simulink model "old_prova_ottimale"  (R2024a)
settings: Solver=VariableStepAuto  StartTime=0.0  StopTime=3000  RelTol=1e-3
undefined symbols (not defined in the file): cp, pitch, TSR
libraries: simulink x4, spsDCMachineLib x1, spsVoltageMeasurementLib x1, sps_lib x1
settings Model: Creator=emanuele  LastModifiedBy=emanuele

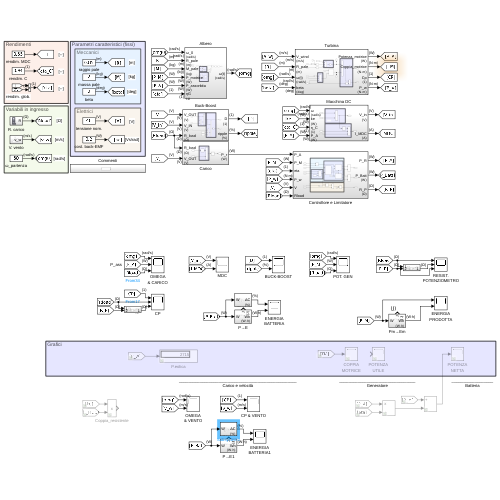
[thumbnail: Simulink's stored preview of the top-level diagram]
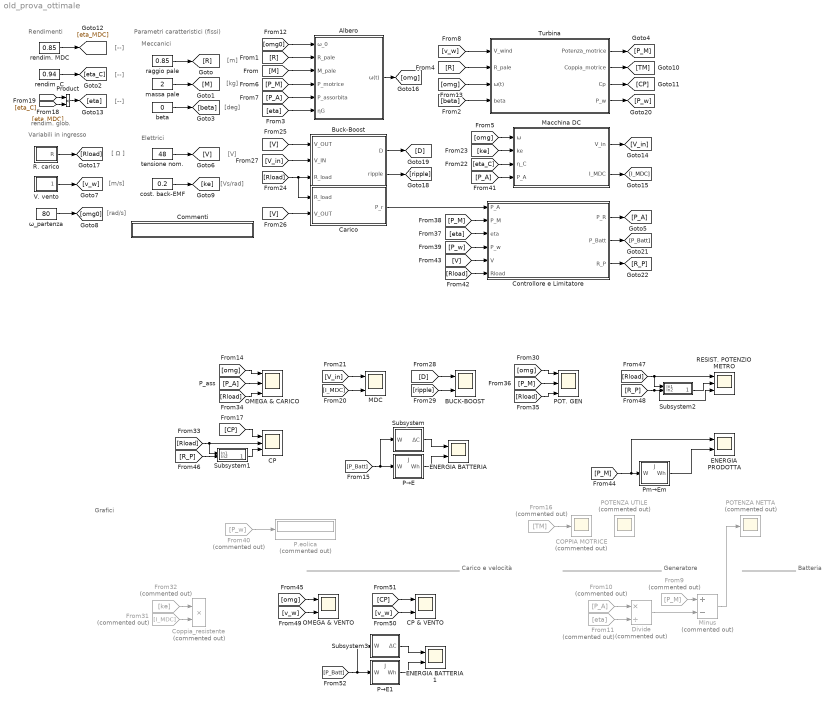
== system old_prova_ottimale ==
  note: rendim. glob.
  note: ___________________________________________________
      | Carico e velocità
  note: Elettrici
  note: Meccanici
  note: Grafici
  note: Variabili in ingresso
  note: [m]
  note: Parametri caratteristici (fissi)
  note: [kg]
  note: [deg]
  note: [ Ω ]
  note: [V]
  note: [m/s]
  note: _________________________________
      | Generatore
  note: __________________
      | Batteria
  note: [rad/s]
  note: Rendimenti
  note: [--]
  note: [--]
  note: [--]
  note: [Vs/rad]
  Albero : Subsystem
  BUCK-BOOST : Scope  NumInputPorts=2
  Buck-Boost : Subsystem
  COPPIA MOTRICE : Scope  Commented=on
  CP : Scope  NumInputPorts=3
  CP & VENTO : Scope  NumInputPorts=2
  Carico : Subsystem
  Commenti : Subsystem
  Controllore e Limitatore : Subsystem
  Coppia_resistente : Product  Commented=on
  Divide : Product  Commented=on  Inputs=*/
  ENERGIA BATTERIA : Scope  NumInputPorts=2
  ENERGIA BATTERIA1 : Scope  NumInputPorts=2
  ENERGIA PRODOTTA : Scope  NumInputPorts=2
  From10 : From  Commented=on  GotoTag=P_A
  From11 : From  Commented=on  GotoTag=eta
  From16 : From  Commented=on  GotoTag=TM
  From31 : From  Commented=on  GotoTag=I_MDC
  From32 : From  Commented=on  GotoTag=ke
  From40 : From  Commented=on  GotoTag=P_w
  From9 : From  Commented=on  GotoTag=P_M
  MDC : Scope  NumInputPorts=2
  Macchina DC : Subsystem
  Minus : Sum  Commented=on  Inputs=+-
  OMEGA & CARICO : Scope  NumInputPorts=3
  OMEGA & VENTO : Scope  NumInputPorts=2
  P.eolica : Display  Commented=on
  POT. GEN : Scope  NumInputPorts=3
  POTENZA NETTA : Scope  Commented=on
  POTENZA UTILE : Scope  Commented=on
  Pm→Em : Subsystem
      settings: PortSchema="{\"entries\":[{\"content\":{\"sides\":[{\"content\":{\"connectorIds\":[\"In1\"]},\"type\":\"ConnectorPlacement.EquallySpacedRectSide\",\"uuid\":\"bcdc19f3-31c9-4960-9b75-9687f3be57dc\"},{\"content\":{\"connectorIds\":[\"Out1\"],\"side\":\"RIGHT\"},\"type\":\"ConnectorPlacement.EquallySpacedRectSide\",\"uuid\":\"6f4d4c58-42a6-48b0-9f12-2aa1dcddf363\"},{\"content\":{\"connectorIds\":[\"Out2\"],\"side\":\"TOP\"},\"type\":\"ConnectorPlacement.EquallySpacedRectSide\",\"uuid\":\"abeed6e6-3a12-4b7a-a1c3-2526a61f695c\"},{\"content\":{\"side\":\"BOTTOM\"},\"type\":\"ConnectorPlacement.EquallySpacedRectSide\",\"uuid\":\"4f3a7421-d380-4df7-a1ed-c17c06ed2066\"}]},\"type\":\"ConnectorPlacement.EquallySpacedConnector\",\"uuid\":\"402fec35-a9bf-47fd-aac8-c2826b6cf801\"}],\"packageUris\":[\"http://schema.mathworks.com/mf0/Connector/R2020b\"],\"version\":\"1.0\"}"
  Product : Product
  P→E : Subsystem
      settings: PortSchema="{\"entries\":[{\"content\":{\"sides\":[{\"content\":{\"connectorIds\":[\"In1\"]},\"type\":\"ConnectorPlacement.EquallySpacedRectSide\",\"uuid\":\"bcdc19f3-31c9-4960-9b75-9687f3be57dc\"},{\"content\":{\"connectorIds\":[\"Out1\"],\"side\":\"RIGHT\"},\"type\":\"ConnectorPlacement.EquallySpacedRectSide\",\"uuid\":\"6f4d4c58-42a6-48b0-9f12-2aa1dcddf363\"},{\"content\":{\"connectorIds\":[\"Out2\"],\"side\":\"TOP\"},\"type\":\"ConnectorPlacement.EquallySpacedRectSide\",\"uuid\":\"abeed6e6-3a12-4b7a-a1c3-2526a61f695c\"},{\"content\":{\"side\":\"BOTTOM\"},\"type\":\"ConnectorPlacement.EquallySpacedRectSide\",\"uuid\":\"4f3a7421-d380-4df7-a1ed-c17c06ed2066\"}]},\"type\":\"ConnectorPlacement.EquallySpacedConnector\",\"uuid\":\"402fec35-a9bf-47fd-aac8-c2826b6cf801\"}],\"packageUris\":[\"http://schema.mathworks.com/mf0/Connector/R2020b\"],\"version\":\"1.0\"}"
  P→E1 : Subsystem
      settings: PortSchema="{\"entries\":[{\"content\":{\"sides\":[{\"content\":{\"connectorIds\":[\"In1\"]},\"type\":\"ConnectorPlacement.EquallySpacedRectSide\",\"uuid\":\"bcdc19f3-31c9-4960-9b75-9687f3be57dc\"},{\"content\":{\"connectorIds\":[\"Out1\"],\"side\":\"RIGHT\"},\"type\":\"ConnectorPlacement.EquallySpacedRectSide\",\"uuid\":\"6f4d4c58-42a6-48b0-9f12-2aa1dcddf363\"},{\"content\":{\"connectorIds\":[\"Out2\"],\"side\":\"TOP\"},\"type\":\"ConnectorPlacement.EquallySpacedRectSide\",\"uuid\":\"abeed6e6-3a12-4b7a-a1c3-2526a61f695c\"},{\"content\":{\"side\":\"BOTTOM\"},\"type\":\"ConnectorPlacement.EquallySpacedRectSide\",\"uuid\":\"4f3a7421-d380-4df7-a1ed-c17c06ed2066\"}]},\"type\":\"ConnectorPlacement.EquallySpacedConnector\",\"uuid\":\"402fec35-a9bf-47fd-aac8-c2826b6cf801\"}],\"packageUris\":[\"http://schema.mathworks.com/mf0/Connector/R2020b\"],\"version\":\"1.0\"}"
  R. carico : Subsystem
  RESIST. POTENZIOMETRO : Scope  NumInputPorts=3
  Subsystem : Subsystem
  Subsystem1 : Subsystem
  Subsystem2 : Subsystem
  Subsystem3 : Subsystem
  Turbina : Subsystem
  V. vento : Subsystem
  beta : Constant  Value=0
  cost. back-EMF : Constant  Value=0.2
  massa pale : Constant  Value=2
  raggio pale : Constant  Value=0.85
  rendim. C : Constant  Value=0.94
  rendim. MDC : Constant  Value=0.85
  tensione nom. : Constant  Value=48
  ω_partenza : Constant  Value=80
  wires:
  raggio pale/1 -> [R]
  massa pale/1 -> [M]
  beta/1 -> [beta]
  [R] -> Albero/2(R_pale)
  [M] -> Albero/3(M_pale)
  [beta] -> Turbina/4(beta)
  [eta] -> Albero/6(ηG)
  [R] -> Turbina/2(R_pale)
  [P_M] -> Albero/4(P_motrice)
  [P_A] -> Albero/5(P_assorbita)
  tensione nom./1 -> [V]
  [P_A] -> OMEGA & CARICO/2
  [v_w] -> Turbina/1(V_wind)
  From9/1 -> Minus/1
  Minus/1 -> POTENZA NETTA/1
  From11/1 -> Divide/2
  From10/1 -> Divide/1
  Divide/1 -> Minus/2
  V. vento/1(v_w) -> [v_w]
  ω_partenza/1 -> [omg0]
  [omg0] -> Albero/1(ω_0)
  Albero/1(ω(t)) -> [omg]
  [omg] -> Macchina DC/1(ω)
  [omg] -> Turbina/3(ω(t))
  [omg] -> OMEGA & CARICO/1
  Turbina/1(Potenza_motrice) -> [P_M]
  [P_Batt] -> Subsystem/1(W), P→E/1(W)
  Turbina/2(Coppia_motrice) -> [TM]
  From16/1 -> COPPIA MOTRICE/1
  Turbina/3(Cp) -> [CP]
  rendim. MDC/1 -> [eta_MDC]
  rendim. C/1 -> [eta_C]
  Product/1 -> [eta]
  [eta_MDC] -> Product/1
  [eta_C] -> Product/2
  [eta_C] -> Macchina DC/3(η_C)
  Macchina DC/1(V_in) -> [V_in]
  Macchina DC/2(I_MDC) -> [I_MDC]
  [V_in] -> MDC/1
  [I_MDC] -> MDC/2
  cost. back-EMF/1 -> [ke]
  [ke] -> Macchina DC/2(ke)
  R. carico/1(R) -> [Rload]
  [Rload] -> Carico/1(R_load), Buck-Boost/3(R_load)
  [V] -> Buck-Boost/1(V_OUT)
  [V] -> Carico/2(V_OUT)
  [V_in] -> Buck-Boost/2(V_IN)
  Buck-Boost/2(ripple) -> [ripple]
  Buck-Boost/1(D) -> [D]
  [D] -> BUCK-BOOST/1
  [ripple] -> BUCK-BOOST/2
  From31/1 -> Coppia_resistente/2
  From32/1 -> Coppia_resistente/1
  [Rload] -> OMEGA & CARICO/3
  [omg] -> POT. GEN/1
  [Rload] -> POT. GEN/3
  [P_M] -> POT. GEN/2
  Carico/1(P_r) -> Controllore e Limitatore/1(P_A)
  Controllore e Limitatore/1(P_R) -> [P_A]
  [P_M] -> Controllore e Limitatore/2(P_M)
  [eta] -> Controllore e Limitatore/3(eta)
  Turbina/4(P_w) -> [P_w]
  [P_w] -> Controllore e Limitatore/4(P_w)
  From40/1 -> P.eolica/1
  Controllore e Limitatore/2(P_Batt) -> [P_Batt]
  [P_A] -> Macchina DC/4(P_A)
  [V] -> Controllore e Limitatore/5(V)
  [Rload] -> Controllore e Limitatore/6(Rload)
  Controllore e Limitatore/3(R_P) -> [R_P]
  [CP] -> CP/1
  [Rload] -> CP/2, Subsystem1/1(In1)
  [R_P] -> Subsystem1/2(In2)
  Subsystem1/1(Out1) -> CP/3
  Subsystem2/1(Out1) -> RESIST. POTENZIOMETRO/2
  [R_P] -> RESIST. POTENZIOMETRO/3, Subsystem2/2(In2)
  [Rload] -> RESIST. POTENZIOMETRO/1, Subsystem2/1(In1)
  [P_M] -> ENERGIA PRODOTTA/1, Pm→Em/1(W)
  Pm→Em/1(Wh) -> ENERGIA PRODOTTA/2
  Subsystem/1(ΔC) -> ENERGIA BATTERIA/1
  P→E/1(Wh) -> ENERGIA BATTERIA/2
  [omg] -> OMEGA & VENTO/1
  [v_w] -> OMEGA & VENTO/2
  [v_w] -> CP & VENTO/2
  [CP] -> CP & VENTO/1
  P→E1/1(Wh) -> ENERGIA BATTERIA1/2
  Subsystem3/1(ΔC) -> ENERGIA BATTERIA1/1
  [P_Batt] -> P→E1/1(W), Subsystem3/1(W)

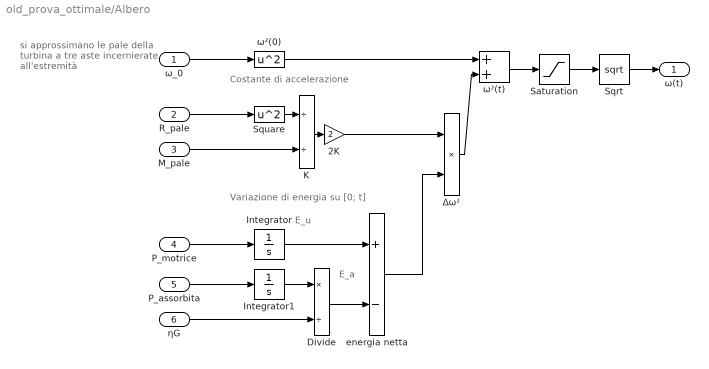
== system old_prova_ottimale/Albero ==
  note: Costante di accelerazione
  note: Variazione di energia su [0; t]
  note: si approssimano le pale
      | della turbina a tre aste
      | incernierate all'estremità
  note: E_a
  note: E_u
  ω_0 : Inport  Unit=rad/s
  R_pale : Inport  Port=2  Unit=m
  M_pale : Inport  Port=3  Unit=kg
  P_motrice : Inport  Port=4  Unit=W
  P_assorbita : Inport  Port=5  Unit=W
  ηG : Inport  Port=6  Unit=1
  2K : Gain  Gain=2
  Divide : Product  Inputs=*/
  Integrator : Integrator
  Integrator1 : Integrator
  K : Product  Inputs=//
  Saturation : Saturate  UpperLimit=10e6  LowerLimit=0
  Sqrt : Sqrt
  Square : Math  Operator=square
  energia netta : Sum  Inputs=+-
  Δω² : Product
  ω²(0) : Math  Operator=square
  ω²(t) : Sum
  ω(t) : Outport  Unit=rad/s
  wires:
  M_pale/1 -> K/2
  K/1 -> 2K/1
  Sqrt/1 -> ω(t)/1
  energia netta/1 -> Δω²/2
  Integrator/1 -> energia netta/1
  R_pale/1 -> Square/1
  P_assorbita/1 -> Integrator1/1
  Integrator1/1 -> Divide/1
  Δω²/1 -> ω²(t)/2
  Square/1 -> K/1
  P_motrice/1 -> Integrator/1
  ω²(0)/1 -> ω²(t)/1
  ω_0/1 -> ω²(0)/1
  ω²(t)/1 -> Saturation/1
  2K/1 -> Δω²/1
  Divide/1 -> energia netta/2
  ηG/1 -> Divide/2
  Saturation/1 -> Sqrt/1

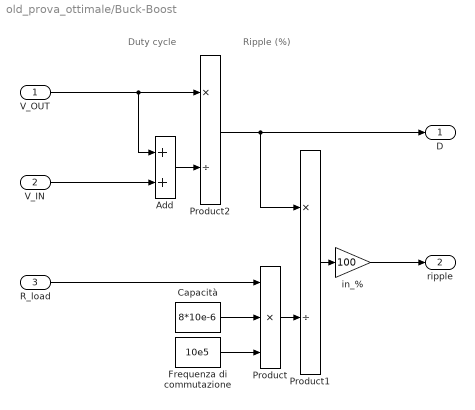
== system old_prova_ottimale/Buck-Boost ==
  note: Duty cycle
  note: Ripple (%)
  V_OUT : Inport  Unit=V
  V_IN : Inport  Port=2  Unit=V
  R_load : Inport  Port=3  Unit=Ω
  Add : Sum
  Capacità : Constant  Value=8*10e-6
  Frequenza di commutazione : Constant  Value=10e5
  Product : Product  Inputs=3
  Product1 : Product  Inputs=*/
  Product2 : Product  Inputs=*/
  in_% : Gain  Gain=100
  D : Outport  Unit=1
  ripple : Outport  Port=2  Unit=%
  wires:
  R_load/1 -> Product/1
  Capacità/1 -> Product/2
  V_IN/1 -> Add/2
  Frequenza di commutazione/1 -> Product/3
  Product/1 -> Product1/2
  V_OUT/1 -> Product2/1, Add/1
  Add/1 -> Product2/2
  Product1/1 -> in_%/1
  in_%/1 -> ripple/1
  Product2/1 -> D/1, Product1/1

== system old_prova_ottimale/Carico ==
  note: Carico
  R_load : Inport  Unit=Ω
  V_OUT : Inport  Port=2  Unit=V
  Product : Product  Inputs=*/
  Saturation : Saturate  UpperLimit=10e6  LowerLimit=0.1
  Square : Math  Operator=square
  P_r : Outport  Unit=W
  wires:
  Square/1 -> Product/1
  R_load/1 -> Product/2
  Product/1 -> Saturation/1
  V_OUT/1 -> Square/1
  Saturation/1 -> P_r/1

== system old_prova_ottimale/Commenti ==
  note: % se omega = 0 → solo P_A
      | % come calcolo il deficit di energia?
  vecchia MDC : Subsystem  Commented=on

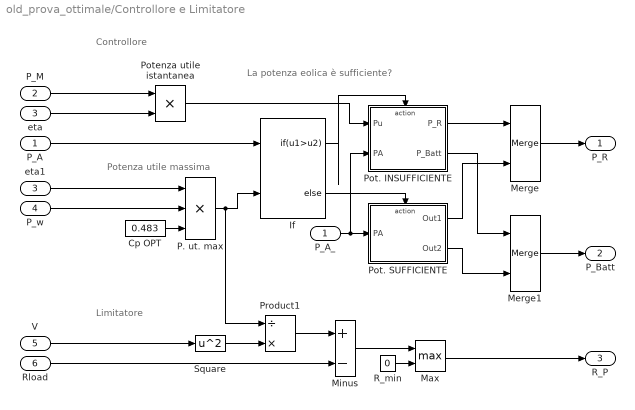
== system old_prova_ottimale/Controllore e Limitatore ==
  note: Limitatore
  note: Controllore
  note: Potenza utile massima
  note: La potenza eolica è sufficiente?
  P_A : Inport
  P_M : Inport  Port=2
  eta : Inport  Port=3
  P_w : Inport  Port=4
  V : Inport  Port=5
  Rload : Inport  Port=6
  Cp OPT : Constant  Value=0.483
  If : If  NumInputs=2  IfExpression=u1>u2
  Max : MinMax  Function=max  Inputs=2
  Merge : Merge
  Merge1 : Merge
  Minus : Sum  Inputs=+-
  P. ut. max : Product  Inputs=3
  P_A_ : InportShadow
  Pot. INSUFFICIENTE : Subsystem  TreatAsAtomicUnit=on
  Pot. SUFFICIENTE : Subsystem  TreatAsAtomicUnit=on
  Potenza utile istantanea : Product
  Product1 : Product  Inputs=/*
  R_min : Constant  Value=0
  Square : Math  Operator=square
  eta1 : InportShadow  Port=3
  P_R : Outport
  P_Batt : Outport  Port=2  Unit=W
  R_P : Outport  Port=3  Unit=Ω
  wires:
  P_M/1 -> Potenza utile istantanea/1
  eta/1 -> Potenza utile istantanea/2
  Pot. SUFFICIENTE/1(Out1) -> Merge/2
  Merge/1 -> P_R/1
  Pot. INSUFFICIENTE/1(P_R) -> Merge/1
  If/2 -> Pot. SUFFICIENTE/Action
  P_A/1 -> If/1
  Potenza utile istantanea/1 -> Pot. INSUFFICIENTE/1(Pu)
  P_A_/1 -> Pot. INSUFFICIENTE/2(PA), Pot. SUFFICIENTE/1(PA)
  If/1 -> Pot. INSUFFICIENTE/Action
  eta1/1 -> P. ut. max/1
  P_w/1 -> P. ut. max/2
  Cp OPT/1 -> P. ut. max/3
  Merge1/1 -> P_Batt/1
  Pot. SUFFICIENTE/2(Out2) -> Merge1/2
  Pot. INSUFFICIENTE/2(P_Batt) -> Merge1/1
  V/1 -> Square/1
  Square/1 -> Product1/2
  Product1/1 -> Minus/1
  Rload/1 -> Minus/2
  Max/1 -> R_P/1
  Minus/1 -> Max/1
  R_min/1 -> Max/2
  P. ut. max/1 -> Product1/1, If/2

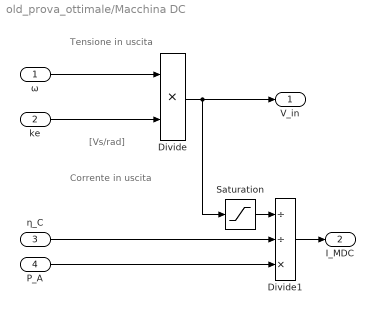
== system old_prova_ottimale/Macchina DC ==
  note: Corrente in uscita
  note: [Vs/rad]
  note: Tensione in uscita
  ω : Inport  Unit=rad/s
  ke : Inport  Port=2  Unit=W
  η_C : Inport  Port=3  Unit=1
  P_A : Inport  Port=4  Unit=W
  Divide : Product
  Divide1 : Product  Inputs=//*
  Saturation : Saturate  UpperLimit=1000  LowerLimit=1
  V_in : Outport  Unit=V
  I_MDC : Outport  Port=2  Unit=A
  wires:
  ke/1 -> Divide/2
  η_C/1 -> Divide1/2
  Saturation/1 -> Divide1/1
  Divide1/1 -> I_MDC/1
  ω/1 -> Divide/1
  Divide/1 -> V_in/1, Saturation/1
  P_A/1 -> Divide1/3

== system old_prova_ottimale/Pm→Em ==
  W : Inport
  J→Wh : Gain  Gain=1/3600
  integrale in dt : Integrator
  Wh : Outport  Unit=W*h
  J : Outport  Port=2  Unit=J
  wires:
  integrale in dt/1 -> J/1, J→Wh/1
  J→Wh/1 -> Wh/1
  W/1 -> integrale in dt/1

== system old_prova_ottimale/P→E ==
  W : Inport
  Gain : Gain  Gain=-1
  J→Wh : Gain  Gain=1/3600
  integrale in dt : Integrator
  Wh : Outport  Unit=W*h
  J : Outport  Port=2  Unit=J
  wires:
  integrale in dt/1 -> Gain/1
  J→Wh/1 -> Wh/1
  W/1 -> integrale in dt/1
  Gain/1 -> J/1, J→Wh/1

== system old_prova_ottimale/P→E1 ==
  W : Inport
  Gain : Gain
  J→Wh : Gain  Gain=1/3600
  integrale in dt : Integrator
  Wh : Outport  Unit=W*h
  J : Outport  Port=2  Unit=J
  wires:
  Gain/1 -> J→Wh/1, J/1
  W/1 -> integrale in dt/1
  J→Wh/1 -> Wh/1
  integrale in dt/1 -> Gain/1

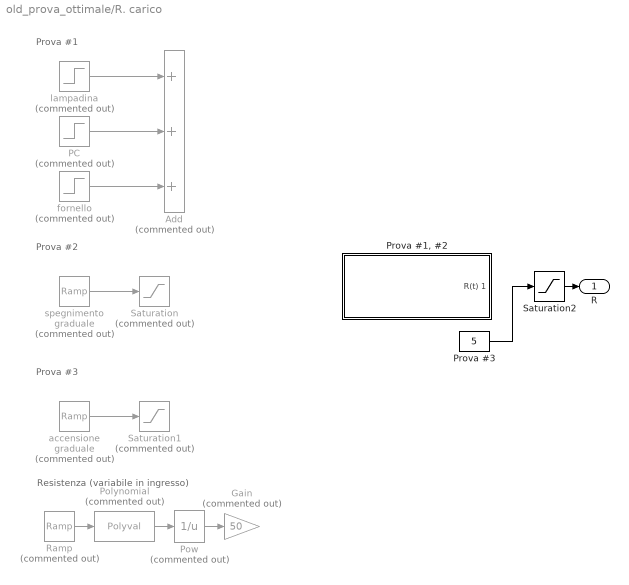
== system old_prova_ottimale/R. carico ==
  note: Prova #1
  note: Prova #2
  note: Prova #3
  note: Resistenza (variabile in ingresso)
  Add : Sum  Commented=on  Inputs=+++
  Gain : Gain  Commented=on  Gain=50
  PC : Step  Commented=on  Time=1200  After=90  SampleTime=0
  Polynomial : Polyval  Commented=on  Coefs=[10e-4 0 0]
  Pow : Math  Commented=on  Operator=reciprocal  SignedPower=on  RndMeth=Zero
  "Prova #1, #2" : Subsystem
  Prova #3 : Constant  Value=5
  Ramp : simulink/Sources/Ramp  Commented=on  slope=0.12  start=100  InitialOutput=0.1
  Saturation : Saturate  Commented=on  UpperLimit=1000  LowerLimit=0
  Saturation1 : Saturate  Commented=on  UpperLimit=200  LowerLimit=0
  Saturation2 : Saturate  UpperLimit=10e6  LowerLimit=0.15
  accensione graduale : simulink/Sources/Ramp  Commented=on  slope=2  start=900  InitialOutput=0
  fornello : Step  Commented=on  Time=1500  After=900  SampleTime=0
  lampadina : Step  Commented=on  Time=900  After=10  SampleTime=0
  spegnimento graduale : simulink/Sources/Ramp  Commented=on  slope=-10  start=900  InitialOutput=1000
  R : Outport
  wires:
  lampadina/1 -> Add/1
  PC/1 -> Add/2
  fornello/1 -> Add/3
  spegnimento graduale/1 -> Saturation/1
  accensione graduale/1 -> Saturation1/1
  Pow/1 -> Gain/1
  Ramp/1 -> Polynomial/1
  Polynomial/1 -> Pow/1
  Saturation2/1 -> R/1
  Prova #3/1 -> Saturation2/1

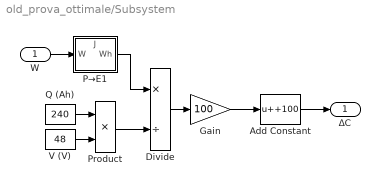
== system old_prova_ottimale/Subsystem ==
  W : Inport
  Add Constant : Bias  Bias=+100  SaturateOnIntegerOverflow=off
  Divide : Product  Inputs=*/
  Gain : Gain  Gain=100
  Product : Product
  P→E1 : Subsystem
      settings: PortSchema="{\"entries\":[{\"content\":{\"sides\":[{\"content\":{\"connectorIds\":[\"In1\"]},\"type\":\"ConnectorPlacement.EquallySpacedRectSide\",\"uuid\":\"bcdc19f3-31c9-4960-9b75-9687f3be57dc\"},{\"content\":{\"connectorIds\":[\"Out1\"],\"side\":\"RIGHT\"},\"type\":\"ConnectorPlacement.EquallySpacedRectSide\",\"uuid\":\"6f4d4c58-42a6-48b0-9f12-2aa1dcddf363\"},{\"content\":{\"connectorIds\":[\"Out2\"],\"side\":\"TOP\"},\"type\":\"ConnectorPlacement.EquallySpacedRectSide\",\"uuid\":\"abeed6e6-3a12-4b7a-a1c3-2526a61f695c\"},{\"content\":{\"side\":\"BOTTOM\"},\"type\":\"ConnectorPlacement.EquallySpacedRectSide\",\"uuid\":\"4f3a7421-d380-4df7-a1ed-c17c06ed2066\"}]},\"type\":\"ConnectorPlacement.EquallySpacedConnector\",\"uuid\":\"402fec35-a9bf-47fd-aac8-c2826b6cf801\"}],\"packageUris\":[\"http://schema.mathworks.com/mf0/Connector/R2020b\"],\"version\":\"1.0\"}"
  Q (Ah) : Constant  Value=240
  V (V) : Constant  Value=48
  ΔC : Outport  Unit=%
  wires:
  W/1 -> P→E1/1(W)
  V (V)/1 -> Product/2
  Q (Ah)/1 -> Product/1
  Product/1 -> Divide/2
  Divide/1 -> Gain/1
  P→E1/1(Wh) -> Divide/1
  Gain/1 -> Add Constant/1
  Add Constant/1 -> ΔC/1

== system old_prova_ottimale/Subsystem1 ==
  In1 : Inport
  In2 : Inport  Port=2
  Add : Sum
  Out1 : Outport  Unit=Ω
  wires:
  Add/1 -> Out1/1
  In2/1 -> Add/2
  In1/1 -> Add/1

== system old_prova_ottimale/Subsystem2 ==
  In1 : Inport
  In2 : Inport  Port=2
  Add : Sum
  Out1 : Outport  Unit=Ω
  wires:
  In1/1 -> Add/1
  In2/1 -> Add/2
  Add/1 -> Out1/1

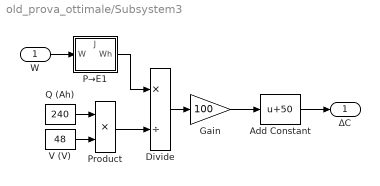
== system old_prova_ottimale/Subsystem3 ==
  W : Inport
  Add Constant : Bias  Bias=50  SaturateOnIntegerOverflow=off
  Divide : Product  Inputs=*/
  Gain : Gain  Gain=100
  Product : Product
  P→E1 : Subsystem
      settings: PortSchema="{\"entries\":[{\"content\":{\"sides\":[{\"content\":{\"connectorIds\":[\"In1\"]},\"type\":\"ConnectorPlacement.EquallySpacedRectSide\",\"uuid\":\"bcdc19f3-31c9-4960-9b75-9687f3be57dc\"},{\"content\":{\"connectorIds\":[\"Out1\"],\"side\":\"RIGHT\"},\"type\":\"ConnectorPlacement.EquallySpacedRectSide\",\"uuid\":\"6f4d4c58-42a6-48b0-9f12-2aa1dcddf363\"},{\"content\":{\"connectorIds\":[\"Out2\"],\"side\":\"TOP\"},\"type\":\"ConnectorPlacement.EquallySpacedRectSide\",\"uuid\":\"abeed6e6-3a12-4b7a-a1c3-2526a61f695c\"},{\"content\":{\"side\":\"BOTTOM\"},\"type\":\"ConnectorPlacement.EquallySpacedRectSide\",\"uuid\":\"4f3a7421-d380-4df7-a1ed-c17c06ed2066\"}]},\"type\":\"ConnectorPlacement.EquallySpacedConnector\",\"uuid\":\"402fec35-a9bf-47fd-aac8-c2826b6cf801\"}],\"packageUris\":[\"http://schema.mathworks.com/mf0/Connector/R2020b\"],\"version\":\"1.0\"}"
  Q (Ah) : Constant  Value=240
  V (V) : Constant  Value=48
  ΔC : Outport  Unit=%
  wires:
  Add Constant/1 -> ΔC/1
  Gain/1 -> Add Constant/1
  P→E1/1(Wh) -> Divide/1
  Divide/1 -> Gain/1
  Product/1 -> Divide/2
  Q (Ah)/1 -> Product/1
  V (V)/1 -> Product/2
  W/1 -> P→E1/1(W)

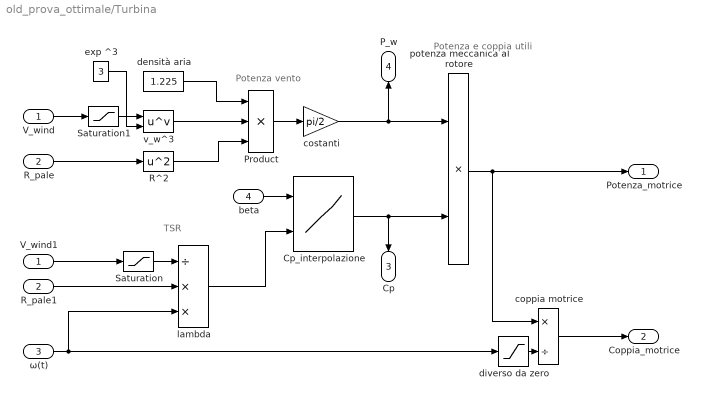
== system old_prova_ottimale/Turbina ==
  note: Potenza e coppia utili
  note: TSR
  note: Potenza vento
  V_wind : Inport  Unit=m/s
  R_pale : Inport  Port=2  Unit=m
  ω(t) : Inport  Port=3  Unit=rad/s
  beta : Inport  Port=4  Unit=deg
  Cp_interpolazione : Lookup_n-D  BreakpointsForDimension1=pitch  BreakpointsForDimension2=TSR  Table=cp  InterpMethod=Cubic spline  InternalRulePriority=Speed  RndMeth=Simplest
      settings: InputPortMap=u0,u1
  Product : Product  Inputs=***
  R^2 : Math  Operator=square
  R_pale1 : InportShadow  Port=2  Unit=m
  Saturation : Saturate  UpperLimit=15  LowerLimit=1
  Saturation1 : Saturate  UpperLimit=15  LowerLimit=1
  V_wind1 : InportShadow  Unit=m/s
  coppia motrice : Product  Inputs=*/
  costanti : Gain  Gain=pi/2
  densità aria : Constant  Value=1.225
  diverso da zero : Saturate  UpperLimit=10e3  LowerLimit=0.1
  exp ^3 : Constant  Value=3
  lambda : Product  Inputs=/**
  potenza meccanica al rotore : Product
  v_w^3 : Math  Operator=pow
  Potenza_motrice : Outport  Unit=W
  Coppia_motrice : Outport  Port=2  Unit=N*m
  Cp : Outport  Port=3  Unit=1
  P_w : Outport  Port=4  Unit=N*m
  wires:
  potenza meccanica al rotore/1 -> coppia motrice/1, Potenza_motrice/1
  R_pale/1 -> R^2/1
  V_wind/1 -> Saturation1/1
  densità aria/1 -> Product/1
  v_w^3/1 -> Product/2
  R^2/1 -> Product/3
  Product/1 -> costanti/1
  Cp_interpolazione/1 -> potenza meccanica al rotore/2, Cp/1
  beta/1 -> Cp_interpolazione/1
  lambda/1 -> Cp_interpolazione/2
  ω(t)/1 -> diverso da zero/1, lambda/3
  diverso da zero/1 -> coppia motrice/2
  coppia motrice/1 -> Coppia_motrice/1
  costanti/1 -> potenza meccanica al rotore/1, P_w/1
  exp ^3/1 -> v_w^3/2
  R_pale1/1 -> lambda/2
  V_wind1/1 -> Saturation/1
  Saturation/1 -> lambda/1
  Saturation1/1 -> v_w^3/1

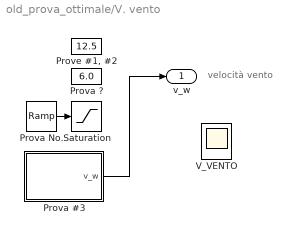
== system old_prova_ottimale/V. vento ==
  note: velocità vento
  Prova #3 : Subsystem
  Prova ? : Constant  Value=6.0
  Prova No. : simulink/Sources/Ramp  slope=0.1  start=900  InitialOutput=2
  "Prove #1, #2" : Constant  Value=12.5
  Saturation : Saturate  UpperLimit=20  LowerLimit=10e-2
  V_VENTO : Scope
  v_w : Outport
  wires:
  Prova No./1 -> Saturation/1
  Prova #3/1(v_w) -> v_w/1

== system old_prova_ottimale/Commenti/vecchia MDC ==
  note: assumo ke = 0.128 Vs/rad
  ω(t) : Inport
  DC Machine : spsDCMachineLib/DC Machine  PresetModel=No  MechanicalLoad=Speed w  FieldType=Permanent magnet  ShowDetailedParameters=on  MeasurementBus=off  RLa="[ 0.6  0.012]"  RLf="[ 240  120]"  Laf=1.8  MachineConstant=Back-emf constant (V/rpm)  Ke=0.05  Kt=1.8  J=1  Bm=0  Tf=0  w0=1  Ifinit=1  TsPowergui=0  TsBlock=-1
  Voltage Measurement : spsVoltageMeasurementLib/Voltage Measurement  PhasorSimulation=off  OutputType=Complex  PSBequivalent=0
  powergui : sps_lib/powergui  Priority=1  SimulationMode=Continuous  SampleTime=50e-6  frequency=60  Iterations=50  frequencyindice=0  Pbase=100e6  ErrMax=1e-4  UnitsV=kV  UnitsW=MW  buscounter=0  FunctionMessages=off  echomessages=off  EnableUseOfTLC=off  CurrentSourceSwitches=off  DisableSnubberDevices=off  DisableRonSwitches=off  DisableVfSwitches=off  DisplayEquations=off  AutomaticDiscreteSolvers=off  SolverType=Tustin/Backward Euler (TBE)  Interpol=off  ExternalGateDelay=off  methode=off  Ts=100  x0status=blocks  SPID=on  SwTol=0  HookPort=off  NonlinearTolerance=1e-4  nMaxIteration=100  ContinueOnMaxIteration=off  RestoreLinks=warning  ResistiveCurrentMeasurement=off  Frange=[0:2:500]  Ylog=off  Xlog=on  ShowGrid=off  save=off  variable=ZData  structure=0  ZoomFFT=off  StartTime=0.0  cycles=1  DisplayStyle=1  fundamental=60  FreqAxis=off  MaxFrequency=1000  frequencyindicesteady=1  RmsSteady=1  display=off
  m : Outport
  V : Outport  Port=2  Unit=V
  wires:
  ω(t)/1 -> DC Machine/1
  DC Machine/1 -> m/1
  Voltage Measurement/1 -> V/1
  connections:
  Voltage Measurement/LConn2 -- DC Machine/RConn1
  DC Machine/LConn1 -- Voltage Measurement/LConn1

== system old_prova_ottimale/Controllore e Limitatore/Pot. INSUFFICIENTE ==
  Pu : Inport
  PA : Inport  Port=2
  Action Port : ActionPort  ActionPortLabel=if(u1>u2)
  Minus : Sum  Inputs=-+
  P_R : Outport
  P_Batt : Outport  Port=2  Unit=W
  wires:
  PA/1 -> Minus/2
  Minus/1 -> P_Batt/1
  Pu/1 -> Minus/1, P_R/1

== system old_prova_ottimale/Controllore e Limitatore/Pot. SUFFICIENTE ==
  PA : Inport
  Action Port : ActionPort  ActionPortLabel=else
  Constant : Constant  Value=0
  Out1 : Outport
  Out2 : Outport  Port=2  Unit=W
  wires:
  PA/1 -> Out1/1
  Constant/1 -> Out2/1

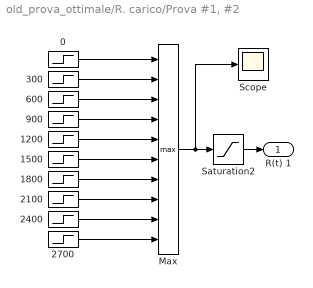
== system old_prova_ottimale/R. carico/Prova #1, #2 ==
  0 : Step  Time=300  Before=100  After=0  SampleTime=0
  1200 : Step  Time=1500  Before=2.8  After=0  SampleTime=0
  1500 : Step  Time=1800  Before=2.6  After=0  SampleTime=0
  1800 : Step  Time=2100  Before=2.4  After=0  SampleTime=0
  2100 : Step  Time=2400  Before=2.2  After=0  SampleTime=0
  2400 : Step  Time=2700  Before=2  After=0  SampleTime=0
  2700 : Step  Time=3000  Before=1.0  After=0  SampleTime=0
  300 : Step  Time=600  Before=10  After=0  SampleTime=0
  600 : Step  Time=900  Before=5  After=0  SampleTime=0
  900 : Step  Time=1200  Before=3  After=0  SampleTime=0
  Max : MinMax  Function=max  Inputs=10
  Saturation2 : Saturate  UpperLimit=10e6  LowerLimit=0.15
  Scope : Scope
  R(t) 1 : Outport
  wires:
  2400/1 -> Max/9
  600/1 -> Max/3
  Max/1 -> Scope/1, Saturation2/1
  1800/1 -> Max/7
  2700/1 -> Max/10
  1500/1 -> Max/6
  1200/1 -> Max/5
  0/1 -> Max/1
  900/1 -> Max/4
  2100/1 -> Max/8
  300/1 -> Max/2
  Saturation2/1 -> R(t) 1/1

== system old_prova_ottimale/Subsystem/P→E1 ==
  W : Inport
  Gain : Gain  Gain=-1
  J→Wh : Gain  Gain=1/3600
  integrale in dt : Integrator
  Wh : Outport  Unit=W*h
  J : Outport  Port=2  Unit=J
  wires:
  Gain/1 -> J→Wh/1, J/1
  W/1 -> integrale in dt/1
  J→Wh/1 -> Wh/1
  integrale in dt/1 -> Gain/1

== system old_prova_ottimale/Subsystem3/P→E1 ==
  W : Inport
  Gain : Gain
  J→Wh : Gain  Gain=1/3600
  integrale in dt : Integrator
  Wh : Outport  Unit=W*h
  J : Outport  Port=2  Unit=J
  wires:
  integrale in dt/1 -> Gain/1
  J→Wh/1 -> Wh/1
  W/1 -> integrale in dt/1
  Gain/1 -> J/1, J→Wh/1

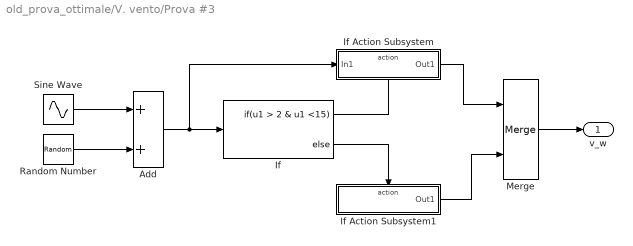
== system old_prova_ottimale/V. vento/Prova #3 ==
  Add : Sum
  If : If  IfExpression=u1 > 2 & u1 <15
  If Action Subsystem : Subsystem  TreatAsAtomicUnit=on
  If Action Subsystem1 : Subsystem  TreatAsAtomicUnit=on
  Merge : Merge
  Random Number : RandomNumber  Variance=2  SampleTime=1
  Sine Wave : Sin  Amplitude=5.5  Bias=8.5  Frequency=2*pi/90  SampleTime=0
  v_w : Outport
  wires:
  If/2 -> If Action Subsystem1/Action
  Add/1 -> If Action Subsystem/1(In1), If/1
  Sine Wave/1 -> Add/1
  Merge/1 -> v_w/1
  Random Number/1 -> Add/2
  If Action Subsystem/1(Out1) -> Merge/1
  If Action Subsystem1/1(Out1) -> Merge/2
  If/1 -> If Action Subsystem/Action

== system old_prova_ottimale/V. vento/Prova #3/If Action Subsystem ==
  In1 : Inport
  Action Port : ActionPort  ActionPortLabel=if(u1 > 2 & u1 <15)
  Out1 : Outport
  wires:
  In1/1 -> Out1/1

== system old_prova_ottimale/V. vento/Prova #3/If Action Subsystem1 ==
  Action Port : ActionPort  ActionPortLabel=else
  Constant : Constant  Value=0
  Out1 : Outport
  wires:
  Constant/1 -> Out1/1
